simulink model "mbd2"  (R2021a)
settings: Solver=VariableStepAuto  StartTime=0.0  StopTime=10.0  RelTol=1e-3
settings Model: Creator=Shereen  LastModifiedBy=Shereen
settings OptimizationCC: DefaultParameterBehavior=Inlined  EnhancedBackFolding=on  PassReuseOutputArgsThreshold=0  OptimizeBlockOrder=speed  DifferentSizesBufferReuse=on  OptimizationCustomize=off
settings DebuggingCC: ParameterTunabilityLossMsg=error
settings HardwareCC: TargetBitPerPointer=64  TargetBitPerSizeT=64  TargetBitPerPtrDiffT=64  TargetLongLongMode=on  TargetIntDivRoundTo=Zero  TargetEndianess=LittleEndian  TargetWordSize=64  TargetHWDeviceType=MATLAB Host  ProdEqTarget=off
settings SFSimCC: MATLABDynamicMemAlloc=off
settings RTWCC: Description=Rapid Simulation Target  SystemTargetFile=rsim.tlc  TemplateMakefile=rsim_default_tmf
settings CodeAppCC: ForceParamTrailComments=on  OperatorAnnotations=on
settings RSimTargetCC: TargetLangStandard=C99 (ISO)

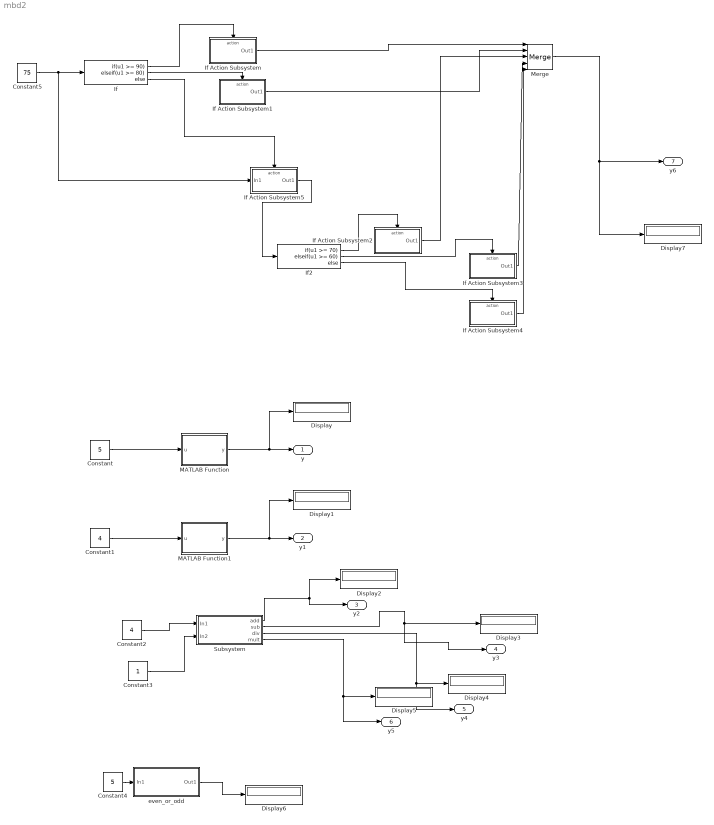
== system mbd2 ==
  Constant : Constant  Value=5
  Constant1 : Constant  Value=4
  Constant2 : Constant  Value=4
  Constant3 : Constant
  Constant4 : Constant  Value=5
  Constant5 : Constant  Value=75
  Display{,1..7} (8 alike) : Display
  If : If  IfExpression=u1 >= 90  ElseIfExpressions=u1 >= 80
  If Action Subsystem : Subsystem  TreatAsAtomicUnit=on
  If Action Subsystem1 : Subsystem  TreatAsAtomicUnit=on
  If Action Subsystem2 : Subsystem  TreatAsAtomicUnit=on
  If Action Subsystem3 : Subsystem  TreatAsAtomicUnit=on
  If Action Subsystem4 : Subsystem  TreatAsAtomicUnit=on
  If Action Subsystem5 : Subsystem  TreatAsAtomicUnit=on
  If2 : If  IfExpression=u1 >= 70  ElseIfExpressions=u1 >= 60
  MATLAB Function : MATLAB Function  TreatAsAtomicUnit=on
  MATLAB Function1 : MATLAB Function  TreatAsAtomicUnit=on
  Merge : Merge  Inputs=5
  Subsystem : Subsystem
  even_or_odd : Subsystem
  y : Outport
  y1 : Outport  Port=2
  y2 : Outport  Port=3
  y3 : Outport  Port=4
  y4 : Outport  Port=5
  y5 : Outport  Port=6
  y6 : Outport  Port=7
  wires:
  Constant/1 -> MATLAB Function/1(u)
  MATLAB Function/1(y) -> Display/1, y/1
  Constant1/1 -> MATLAB Function1/1(u)
  MATLAB Function1/1(y) -> Display1/1, y1/1
  Constant2/1 -> Subsystem/1(In1)
  Subsystem/1(add) -> y2/1, Display2/1
  Constant3/1 -> Subsystem/2(In2)
  Subsystem/2(sub) -> y3/1, Display3/1
  Subsystem/3(div) -> y4/1, Display4/1
  Subsystem/4(mult) -> y5/1, Display5/1
  Constant4/1 -> even_or_odd/1(In1)
  even_or_odd/1(Out1) -> Display6/1
  If/3 -> If Action Subsystem5/Action
  If Action Subsystem5/1(Out1) -> If2/1
  If/1 -> If Action Subsystem/Action
  If2/1 -> If Action Subsystem2/Action
  If2/2 -> If Action Subsystem3/Action
  If2/3 -> If Action Subsystem4/Action
  If Action Subsystem4/1(Out1) -> Merge/5
  If Action Subsystem3/1(Out1) -> Merge/4
  If Action Subsystem2/1(Out1) -> Merge/3
  If Action Subsystem1/1(Out1) -> Merge/2
  If Action Subsystem/1(Out1) -> Merge/1
  Constant5/1 -> If Action Subsystem5/1(In1), If/1
  Merge/1 -> y6/1, Display7/1
  If/2 -> If Action Subsystem1/Action

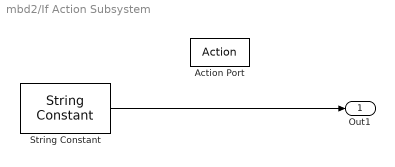
== system mbd2/If Action Subsystem ==
  Action Port : ActionPort  ActionPortLabel=if(u1 >= 90)
  String Constant : StringConstant  String="\"A\""
  Out1 : Outport
  wires:
  String Constant/1 -> Out1/1

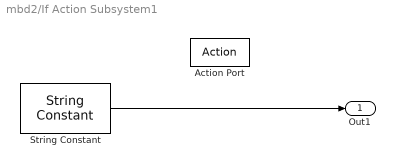
== system mbd2/If Action Subsystem1 ==
  Action Port : ActionPort  ActionPortLabel=elseif(u1 >= 80)
  String Constant : StringConstant  String="\"B\""
  Out1 : Outport
  wires:
  String Constant/1 -> Out1/1

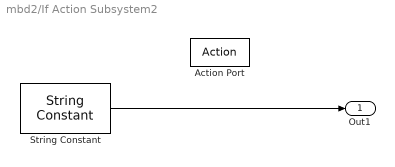
== system mbd2/If Action Subsystem2 ==
  Action Port : ActionPort  ActionPortLabel=if(u1 >= 70)
  String Constant : StringConstant  String="\"C\""
  Out1 : Outport
  wires:
  String Constant/1 -> Out1/1

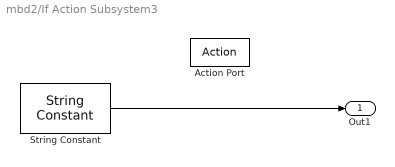
== system mbd2/If Action Subsystem3 ==
  Action Port : ActionPort  ActionPortLabel=elseif(u1 >= 60)
  String Constant : StringConstant  String="\"D\""
  Out1 : Outport
  wires:
  String Constant/1 -> Out1/1

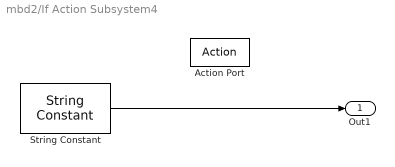
== system mbd2/If Action Subsystem4 ==
  Action Port : ActionPort  ActionPortLabel=else
  String Constant : StringConstant  String="\"F\""
  Out1 : Outport
  wires:
  String Constant/1 -> Out1/1

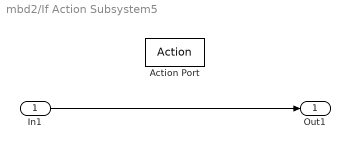
== system mbd2/If Action Subsystem5 ==
  In1 : Inport
  Action Port : ActionPort  ActionPortLabel=else
  Out1 : Outport
  wires:
  In1/1 -> Out1/1

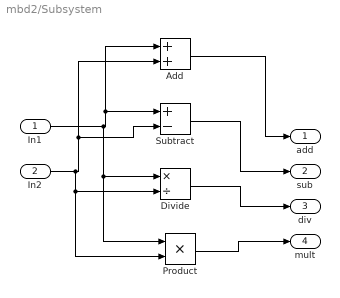
== system mbd2/Subsystem ==
  In1 : Inport
  In2 : Inport  Port=2
  Add : Sum
  Divide : Product  Inputs=*/
  Product : Product
  Subtract : Sum  Inputs=+-
  add : Outport
  sub : Outport  Port=2
  div : Outport  Port=3
  mult : Outport  Port=4
  wires:
  Product/1 -> mult/1
  Divide/1 -> div/1
  Subtract/1 -> sub/1
  Add/1 -> add/1
  In1/1 -> Product/1, Divide/1, Subtract/1, Add/1
  In2/1 -> Product/2, Divide/2, Subtract/2, Add/2

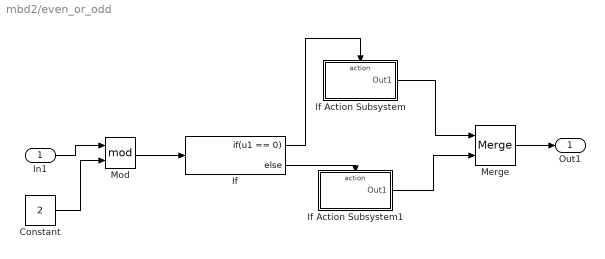
== system mbd2/even_or_odd ==
  In1 : Inport
  Constant : Constant  Value=2
  If : If  IfExpression=u1 == 0
  If Action Subsystem : Subsystem  TreatAsAtomicUnit=on
  If Action Subsystem1 : Subsystem  TreatAsAtomicUnit=on
  Merge : Merge
  Mod : Math  Operator=mod  SaturateOnIntegerOverflow=on
  Out1 : Outport
  wires:
  In1/1 -> Mod/1
  Constant/1 -> Mod/2
  Mod/1 -> If/1
  Merge/1 -> Out1/1
  If Action Subsystem/1(Out1) -> Merge/1
  If/1 -> If Action Subsystem/Action
  If/2 -> If Action Subsystem1/Action
  If Action Subsystem1/1(Out1) -> Merge/2

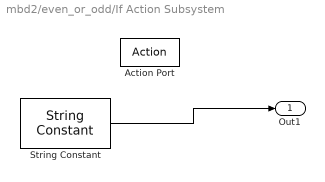
== system mbd2/even_or_odd/If Action Subsystem ==
  Action Port : ActionPort  ActionPortLabel=if(u1 == 0)
  String Constant : StringConstant  String="\"even\""
  Out1 : Outport
  wires:
  String Constant/1 -> Out1/1

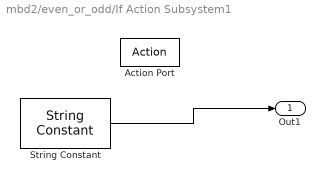
== system mbd2/even_or_odd/If Action Subsystem1 ==
  Action Port : ActionPort  ActionPortLabel=else
  String Constant : StringConstant  String="\"odd\""
  Out1 : Outport
  wires:
  String Constant/1 -> Out1/1

== matlab function mbd2/MATLAB Function ==
  data: u input; y output
function y = fcn(u)
    y=1;
    for i=1:u
        y=y*i;
    end
end

== matlab function mbd2/MATLAB Function1 ==
  data: u input; y output
function y = fcn(u)
    y = 1;
    i = 1;
    while i <= u
        y = y * i;
        i = i + 1;
    end
end
